simulink model "raspberrypi_SPI_EEPROM"  (R2018b)
settings: Solver=FixedStepAuto  StartTime=0.0  StopTime=inf  RelTol=1e-3
libraries: raspberrypilib x3, realtime_examples_misc x1
settings Model: SimulationMode=external  ExtModeTrigDuration=2  Creator=The MathWorks, Inc.  LastModifiedBy=The MathWorks, Inc.
settings SolverCC: PositivePriorityOrder=on
settings DataIOCC: LimitDataPoints=on
settings OptimizationCC: BlockReduction=off  LifeSpan=1  MaxStackSize=64
settings DebuggingCC: AllowSymbolicDim=off  SFUnexpectedBacktrackingDiag=warning  SFNoUnconditionalDefaultTransitionDiag=warning  SFExecutionAtInitializationDiag=none
settings HardwareCC: ProdBitPerPointer=32  ProdBitPerSizeT=32  ProdBitPerPtrDiffT=32  ProdLargestAtomicInteger=Long  ProdLargestAtomicFloat=Double  ProdWordSize=32  ProdHWDeviceType=ARM Compatible->ARM Cortex  UseEmbeddedCoderFeatures=off  UseSimulinkCoderFeatures=off
settings ModelReferenceCC: PropagateSignalLabelsOutOfModel=off
settings SFSimCC: SimUseLocalCustomCode=off
settings RTWCC: SystemTargetFile=ert.tlc  HardwareBoard=Raspberry Pi  TemplateMakefile=ert_default_tmf  RTWUseLocalCustomCode=off  Toolchain=GNU GCC Raspberry Pi  BuildConfiguration=Faster Runs
settings CodeAppCC: StateflowObjectComments=on
settings ERTTargetCC: MultiwordLength=2048  ERTCustomFileBanners=off  SupportContinuousTime=on  SupportNonInlinedSFcns=on  RemoveResetFunc=off  SupportVariableSizeSignals=on  ModelStepFunctionPrototypeControlCompliant=off  ConvertIfToSwitch=off  SuppressUnreachableDefaultCases=off
settings ConfigComp: CovMetricSettings=dw  CovHtmlReporting=on  CovSaveCumulativeToWorkspaceVar=on  CovSaveSingleToWorkspaceVar=on  CovExternalEMLEnable=off

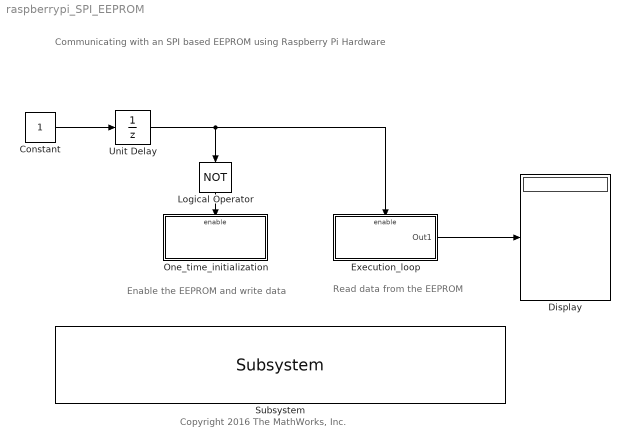
== system raspberrypi_SPI_EEPROM ==
  note: Read data from the EEPROM
  note: Enable the EEPROM and write data
  note: Communicating with an SPI based EEPROM
      | using Raspberry Pi Hardware
  note: Copyright 2016 The MathWorks, Inc.
  Constant : Constant  OutDataTypeStr=boolean  SampleTime=0.1
  Display : Display
  Execution_loop : Subsystem  TreatAsAtomicUnit=on
  Logical Operator : Logic  Operator=NOT  AllPortsSameDT=off  OutDataTypeStr=boolean
  One_time_initialization : Subsystem  TreatAsAtomicUnit=on
  Subsystem : realtime_examples_misc/Subsystem  SystemSampleTime=-1
  Unit Delay : UnitDelay  SampleTime=-1
  wires:
  Constant/1 -> Unit Delay/1
  Unit Delay/1 -> Execution_loop/Enable, Logical Operator/1
  Logical Operator/1 -> One_time_initialization/Enable
  Execution_loop/1(Out1) -> Display/1

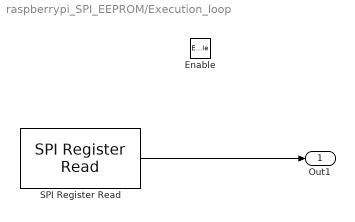
== system raspberrypi_SPI_EEPROM/Execution_loop ==
  Enable : EnablePort  StatesWhenEnabling=reset
  SPI Register Read : raspberrypilib/SPI Register Read  BoardProperty=Pi 3 Model B  SPIModule=uint32(0)  Mode=Master  BusSpeed=1000000  Pin=SPI0_CE0  FirstBitToTransfer=Most significant bit (MSB)  ClockMode=0  BlockFunction=Read  RegisterAddress=[3 0 10]  OutputDataType=int8  OutputDataLength=5  SampleTime=0.1
      settings: SourceProductName=Simulink Support Package for Raspberry Pi Hardware  SourceProductBaseCode=RASPPI
  Out1 : Outport  InitialOutput=0
  wires:
  SPI Register Read/1 -> Out1/1

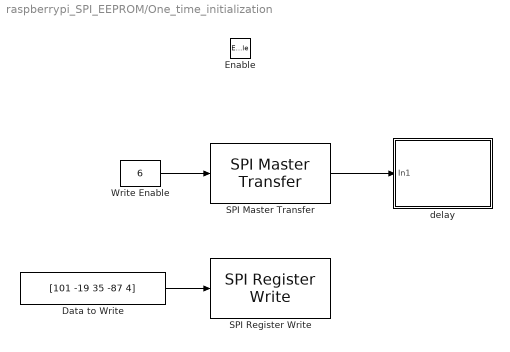
== system raspberrypi_SPI_EEPROM/One_time_initialization ==
  Enable : EnablePort  StatesWhenEnabling=reset
  Data to Write : Constant  Value=[101 -19 35 -87 4]  OutDataTypeStr=int8  SampleTime=0.1
  SPI Master Transfer : raspberrypilib/SPI Master Transfer  BoardProperty=Pi 3 Model B  SPIModule=uint32(0)  Mode=Master  BusSpeed=1000000  Pin=SPI0_CE0  FirstBitToTransfer=Most significant bit (MSB)  ClockMode=0  BlockFunction=Transfer  RegisterAddress=0  OutputDataType=int8  OutputDataLength=1
      settings: SourceProductName=Simulink Support Package for Raspberry Pi Hardware  SourceProductBaseCode=RASPPI
  SPI Register Write : raspberrypilib/SPI Register Write  Priority=6  BoardProperty=Pi 3 Model B  SPIModule=uint32(0)  Mode=Master  BusSpeed=1000000  Pin=SPI0_CE0  FirstBitToTransfer=Most significant bit (MSB)  ClockMode=0  BlockFunction=Write  RegisterAddress=[2 0 10]  OutputDataType=int8  OutputDataLength=1
      settings: AttributesFormatString=Priority=%<Priority>  SourceProductName=Simulink Support Package for Raspberry Pi Hardware  SourceProductBaseCode=RASPPI
  Write Enable : Constant  Value=6  OutDataTypeStr=uint8  SampleTime=0.1
  delay : Subsystem  Priority=1
      settings: AttributesFormatString=Priority=%<Priority>
  wires:
  Write Enable/1 -> SPI Master Transfer/1
  SPI Master Transfer/1 -> delay/1(In1)
  Data to Write/1 -> SPI Register Write/1

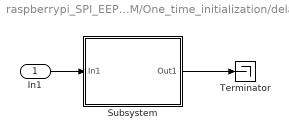
== system raspberrypi_SPI_EEPROM/One_time_initialization/delay ==
  In1 : Inport
  Subsystem : Subsystem
  Terminator : Terminator
  wires:
  Subsystem/1(Out1) -> Terminator/1
  In1/1 -> Subsystem/1(In1)

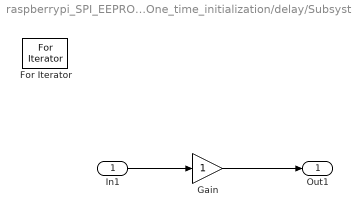
== system raspberrypi_SPI_EEPROM/One_time_initialization/delay/Subsystem ==
  In1 : Inport
  For Iterator : ForIterator  IterationLimit=10000  ShowIterationPort=off  IndexMode=Zero-based
  Gain : Gain  OutDataTypeStr=Inherit: Same as input  ParamDataTypeStr=Inherit: Same as input
  Out1 : Outport
  wires:
  In1/1 -> Gain/1
  Gain/1 -> Out1/1
